simulink model "UaUb"  (Simulink 4.00)
settings: Solver=ode45  StartTime=0.0  StopTime=10.0  RelTol=1e-3
settings Model: BlockReductionOpt=off

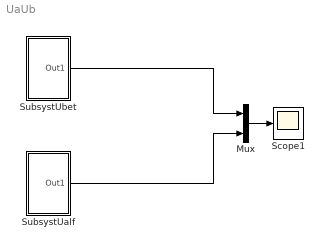
== system UaUb ==
  Mux : Mux  Inputs=2
  Scope1 : Scope
      settings: TimeRange=10  YMin=-1  YMax=1  SaveToWorkspace=off  LimitDataPoints=on  MaxDataPoints=5000
  SubsystUalf : Subsystem
      settings: RTWFcnNameOpts=Auto  RTWFileNameOpts=Auto
  SubsystUbet : Subsystem
      settings: RTWFcnNameOpts=Auto  RTWFileNameOpts=Auto
  wires:
  SubsystUbet/1(Out1) -> Mux/1
  SubsystUalf/1(Out1) -> Mux/2
  Mux/1 -> Scope1/1

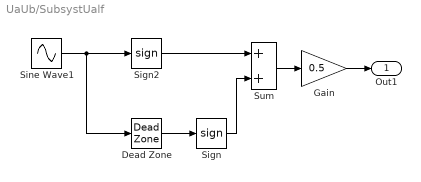
== system UaUb/SubsystUalf ==
  Dead Zone : DeadZone  LowerValue=-0.866  UpperValue=0.866  SaturateOnIntegerOverflow=on  LinearizeAsGain=on
  Gain : Gain  Gain=0.5  Multiplication=Element-wise(K.*u)  SaturateOnIntegerOverflow=on
  Sign : Signum
  Sign2 : Signum
  Sine Wave1 : Sin  Amplitude=1  Frequency=1  Phase=0  SampleTime=0
  Sum : Sum  Inputs=++  SaturateOnIntegerOverflow=on
  Out1 : Outport  Port=1
  wires:
  Sine Wave1/1 -> Sign2/1, Dead Zone/1
  Sign2/1 -> Sum/1
  Dead Zone/1 -> Sign/1
  Sign/1 -> Sum/2
  Sum/1 -> Gain/1
  Gain/1 -> Out1/1

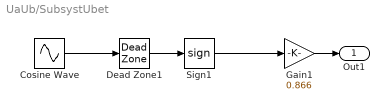
== system UaUb/SubsystUbet ==
  Cosine Wave : Sin  Amplitude=1  Frequency=1  Phase=pi/2  SampleTime=0
  Dead Zone1 : DeadZone  LowerValue=-0.5  UpperValue=0.5  SaturateOnIntegerOverflow=on  LinearizeAsGain=on
  Gain1 : Gain  Gain=0.866  Multiplication=Element-wise(K.*u)  SaturateOnIntegerOverflow=on
  Sign1 : Signum
  Out1 : Outport  Port=1
  wires:
  Cosine Wave/1 -> Dead Zone1/1
  Dead Zone1/1 -> Sign1/1
  Sign1/1 -> Gain1/1
  Gain1/1 -> Out1/1
